simulink model "RegulatorGMK"  (R2020b)
settings: Solver=VariableStepAuto  StartTime=0.0  StopTime=50.0  RelTol=1e-3
settings Model: Creator=user  LastModifiedBy=user

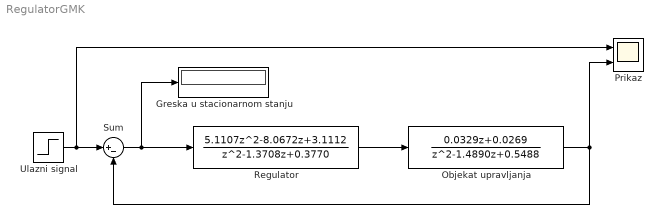
== system RegulatorGMK ==
  Greska u stacionarnom stanju : Display
  Objekat upravljanja : DiscreteTransferFcn  Numerator=[0.0329 0.0269]  Denominator=[1 -1.4890 0.5488]  SampleTime=1
  Prikaz : Scope  NumInputPorts=2
  Regulator : DiscreteTransferFcn  Numerator=[5.1107 -8.0672 3.1112]  Denominator=[1 -1.3708 0.3770]  SampleTime=1
  Sum : Sum  Inputs=|+-
  Ulazni signal : Step  SampleTime=0
  wires:
  Regulator/1 -> Objekat upravljanja/1
  Objekat upravljanja/1 -> Sum/2, Prikaz/2
  Sum/1 -> Regulator/1, Greska u stacionarnom stanju/1
  Ulazni signal/1 -> Sum/1, Prikaz/1
